simulink model "add_test"  (R2021b)
settings: Solver=VariableStepAuto  StartTime=0.0  StopTime=2  MaxStep=1e-8  RelTol=1e-3
undefined symbols (not defined in the file or in its folder): DiscIntNeverNeededParam
libraries: spspowerguiLib x1
settings Model: Creator=phddk  LastModifiedBy=phddk

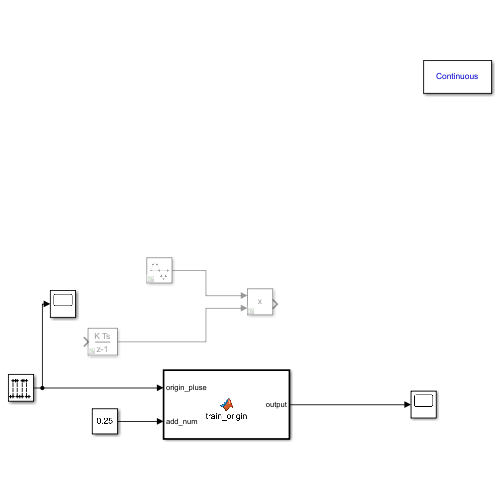
[thumbnail: Simulink's stored preview of the top-level diagram]
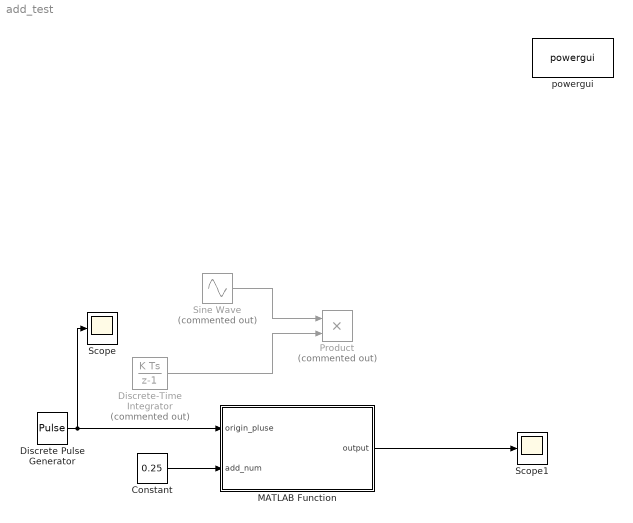
== system add_test ==
  Constant : Constant  Value=0.25
  Discrete Pulse Generator : DiscretePulseGenerator  Period=100  PulseWidth=50  SampleTime=0.001
  Discrete-Time Integrator : DiscreteIntegrator  Commented=on  SampleTime=-1  OutMin=[0]  OutMax=[7]  ICPrevOutput=DiscIntNeverNeededParam  ICPrevScaledInput=DiscIntNeverNeededParam
  MATLAB Function : MATLAB Function  TreatAsAtomicUnit=on
  Product : Product  Commented=on
  Scope : Scope
  Scope1 : Scope
  Sine Wave : Sin  Commented=on  SineType=Sample based  Samples=255  SampleTime=5e-5
  powergui : spspowerguiLib/powergui  Priority=1  SimulationMode=Continuous  SampleTime=50e-6  frequency=60  Iterations=50  frequencyindice=60  Pbase=100e6  ErrMax=1e-4  UnitsV=kV  UnitsW=MW  buscounter=0  FunctionMessages=off  echomessages=off  EnableUseOfTLC=off  CurrentSourceSwitches=off  DisableSnubberDevices=off  DisableRonSwitches=off  DisableVfSwitches=off  DisplayEquations=off  AutomaticDiscreteSolvers=off  SolverType=Tustin/Backward Euler (TBE)  Interpol=off  ExternalGateDelay=off  methode=off  Ts=100  x0status=blocks  SPID=on  SwTol=0  HookPort=off  NonlinearTolerance=1e-4  nMaxIteration=100  ContinueOnMaxIteration=off  RestoreLinks=warning  ResistiveCurrentMeasurement=off  Frange=[0:2:500]  Ylog=off  Xlog=on  ShowGrid=off  save=off  variable=ZData  structure=0  ZoomFFT=off  StartTime=0.0  cycles=1  DisplayStyle=1  fundamental=60  FreqAxis=off  MaxFrequency=1000  frequencyindicesteady=1  RmsSteady=1  display=off
  wires:
  Sine Wave/1 -> Product/1
  Discrete-Time Integrator/1 -> Product/2
  Discrete Pulse Generator/1 -> MATLAB Function/1(origin_pluse), Scope/1
  MATLAB Function/1(output) -> Scope1/1
  Constant/1 -> MATLAB Function/2(add_num)

== matlab function add_test/MATLAB Function ==
  data: origin_pluse input; output output; add_num input
function output  = train_origin(origin_pluse,add_num)

persistent sum_pluse
persistent flag_now
persistent flag_sum

if(isempty(sum_pluse))
    sum_pluse=0;
    flag_now=0;
    flag_sum=0;
end
if (origin_pluse == 1 && flag_now == 0)
    flag_now = 1;
end

if (origin_pluse == 0 && flag_now == 1)
    flag_now = 0;
    flag_sum = 0;
end

if(flag_now == 1 && flag_sum == 0)
    flag_sum = 1;
    sum_pluse = sum_pluse + add_num;
end

output = sum_pluse;
